simulink model "SSBSC_SIM"  (R2024a)
settings: Solver=VariableStepAuto  StartTime=0.0  StopTime=1  RelTol=1e-3
libraries: dspfdesign x2
settings Model: Creator=vnrvjiet  LastModifiedBy=adity
settings SolverCC: AlgebraicLoopSolver=TrustRegion
settings DataIOCC: ReturnWorkspaceOutputs=off
settings DebuggingCC: UnconnectedInputMsg=warning  UnconnectedOutputMsg=warning  UnconnectedLineMsg=warning  ArithmeticOperatorsInVariantConditions=warning
settings ModelReferenceCC: EnableRefExpFcnMdlSchedulingChecks=on
settings SFSimCC: SimUseLocalCustomCode=off  CustomCodeUndefinedFunction=UseInterfaceOnly
settings RTWCC: RTWUseLocalCustomCode=off  GPUComputeCapability=3.5

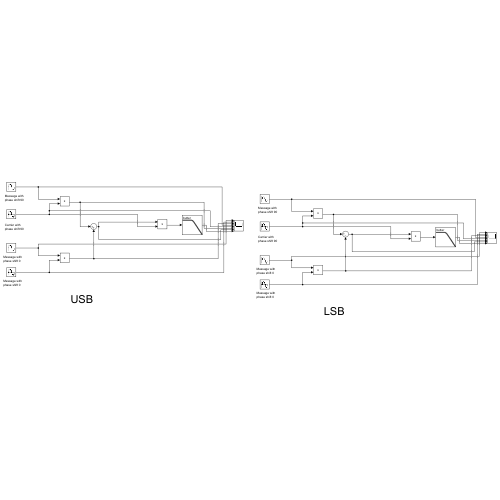
[thumbnail: Simulink's stored preview of the top-level diagram]
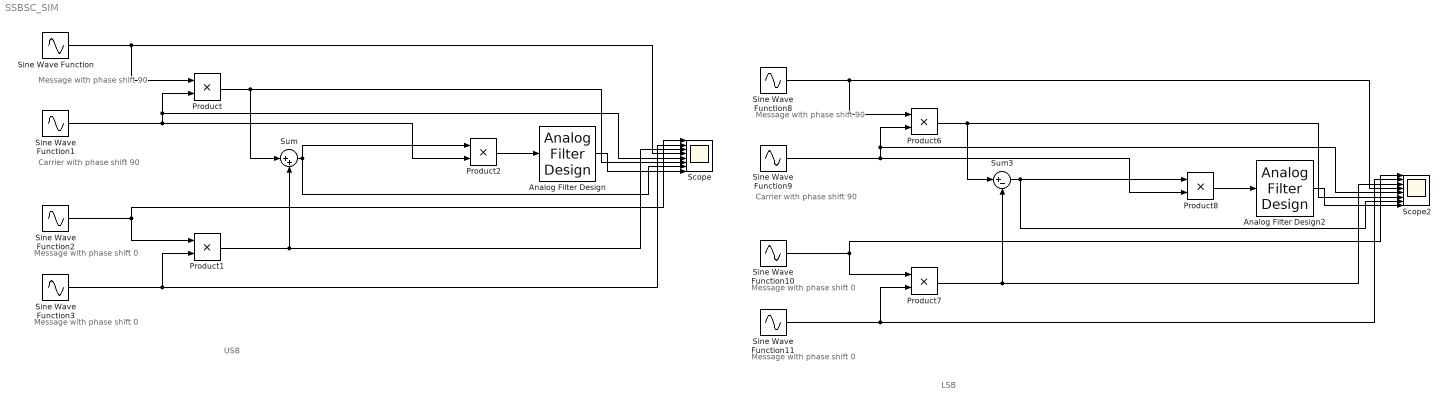
== system SSBSC_SIM ==
  note: Message with
      | phase shift 90
  note: Carrier with
      | phase shift 90
  note: Message with
      | phase shift 0
  note: Message with
      | phase shift 0
  note: USB
  note: Message with
      | phase shift 0
  note: Message with
      | phase shift 90
  note: Carrier with
      | phase shift 90
  note: LSB
  note: Message with
      | phase shift 0
  Analog Filter Design : dspfdesign/Analog Filter Design  method=Butterworth  filttype=Lowpass  N=5  Wlo=2*pi*10  Whi=80  Rp=2  Rs=40
  Analog Filter Design2 : dspfdesign/Analog Filter Design  method=Butterworth  filttype=Lowpass  N=5  Wlo=2*pi*10  Whi=80  Rp=2  Rs=40
  Product{,1..2,6..8} (6 alike) : Product
  Scope : Scope  NumInputPorts=8
  Scope2 : Scope  NumInputPorts=8
  Sine Wave Function : Sin  Frequency=2*pi*10  Phase=pi/2  SampleTime=1/10000
  Sine Wave Function1 : Sin  Frequency=2*pi*100  Phase=pi/2  SampleTime=1/10000
  Sine Wave Function10 : Sin  Frequency=2*pi*10  SampleTime=1/10000
  Sine Wave Function11 : Sin  Frequency=2*pi*100  SampleTime=1/10000
  Sine Wave Function2 : Sin  Frequency=2*pi*10  SampleTime=1/10000
  Sine Wave Function3 : Sin  Frequency=2*pi*100  SampleTime=1/10000
  Sine Wave Function8 : Sin  Frequency=2*pi*10  Phase=pi/2  SampleTime=1/10000
  Sine Wave Function9 : Sin  Frequency=2*pi*100  Phase=pi/2  SampleTime=1/10000
  Sum : Sum  Inputs=|++
  Sum3 : Sum  Inputs=|+-
  wires:
  Sine Wave Function1/1 -> Scope/5, Product/2, Product2/2
  Sine Wave Function2/1 -> Scope/1, Product1/1
  Sine Wave Function3/1 -> Scope/2, Product1/2
  Product/1 -> Scope/6, Sum/1
  Product1/1 -> Scope/3, Sum/2
  Sine Wave Function/1 -> Scope/4, Product/1
  Sum/1 -> Scope/7, Product2/1
  Product2/1 -> Analog Filter Design/1
  Analog Filter Design/1 -> Scope/8
  Sine Wave Function8/1 -> Scope2/4, Product6/1
  Sine Wave Function11/1 -> Scope2/2, Product7/2
  Sum3/1 -> Scope2/7, Product8/1
  Product8/1 -> Analog Filter Design2/1
  Sine Wave Function10/1 -> Scope2/1, Product7/1
  Sine Wave Function9/1 -> Scope2/5, Product6/2, Product8/2
  Product6/1 -> Scope2/6, Sum3/1
  Analog Filter Design2/1 -> Scope2/8
  Product7/1 -> Scope2/3, Sum3/2
